simulink model "Simulink_Lab_7"  (R2025a)
settings: Solver=VariableStepAuto  StartTime=0.0  StopTime=20.0  RelTol=1e-3
libraries: spsDCMachineLib x1, spsDCVoltageSourceLib x1, sps_lib x1
settings Model: Creator=088a2  LastModifiedBy=088a2

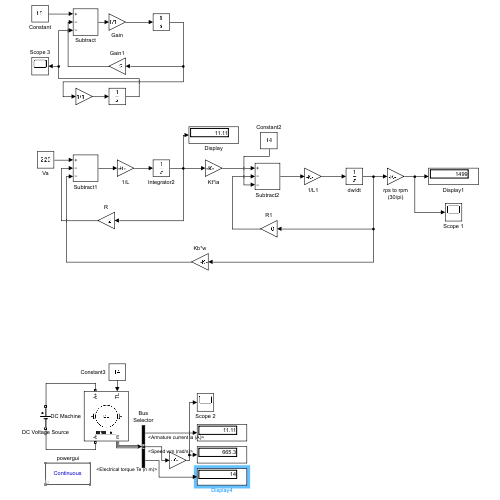
[thumbnail: Simulink's stored preview of the top-level diagram]
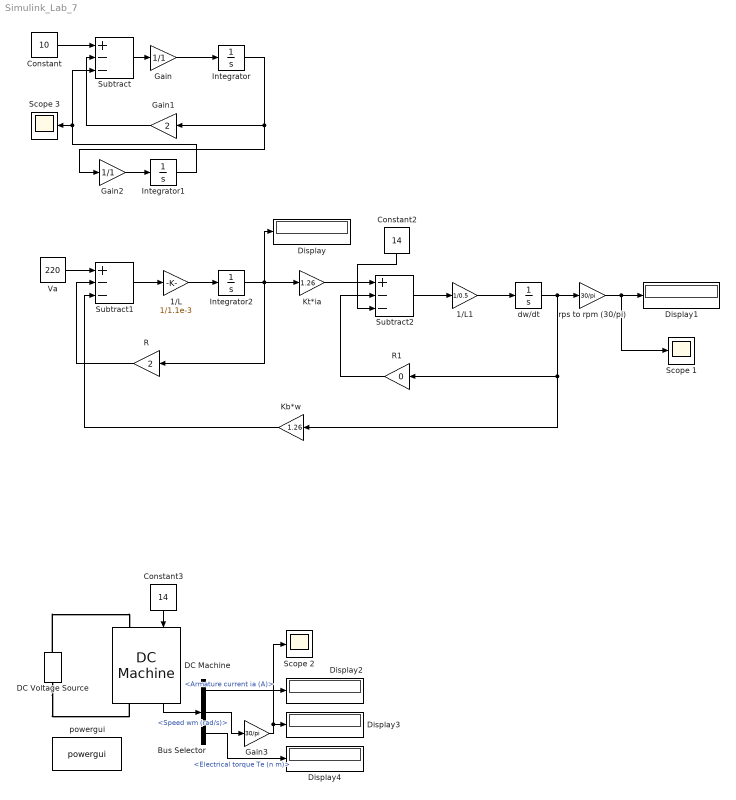
== system Simulink_Lab_7 ==
  1/L : Gain  Gain=1/1.1e-3
  1/L1 : Gain  Gain=1/0.5
  Bus Selector : BusSelector  OutputSignals=Armature current ia (A),Speed wm (rad/s),Electrical torque Te (n m)
  Constant : Constant  Value=10
  Constant2 : Constant  Value=14
  Constant3 : Constant  Value=14
  DC Machine : spsDCMachineLib/DC Machine  PresetModel=No  MechanicalLoad=Torque TL  FieldType=Permanent magnet  ShowDetailedParameters=on  MeasurementBus=off  RLa="[ 2  0.0011]"  RLf="[ 240  120]"  Laf=1.8  MachineConstant=Torque constant (N.m/A)  Ke=1.8  Kt=1.26  J=0.05  Bm=0  Tf=0  w0=1  Ifinit=1  TsPowergui=0  TsBlock=-1
  DC Voltage Source : spsDCVoltageSourceLib/DC Voltage Source  Amplitude=110  Measurements=None
  Display{,1..4} (5 alike) : Display
  Gain : Gain  Gain=1/1
  Gain1 : Gain  Gain=2
  Gain2 : Gain  Gain=1/1
  Gain3 : Gain  Gain=30/pi
  Integrator : Integrator
  Integrator1 : Integrator
  Integrator2 : Integrator
  Kb*w : Gain  Gain=1.26
  Kt*ia : Gain  Gain=1.26
  R : Gain  Gain=2
  R1 : Gain  Gain=0
  Scope 1 : Scope
      settings: Title=230929228_Mrinal_Kumar  ActiveDisplayYMinimum=-187.37365805398784  ActiveDisplayYMaximum=1686.2872524111651  YLabel=Voltage (V)
  Scope 2 : Scope
      settings: Title=230929228_Mrinal_Kumar  ActiveDisplayYMinimum=-72.596030383648909  ActiveDisplayYMaximum=747.24093799551156  YLabel=Voltage (V)
  Scope 3 : Scope
      settings: Title=230929228_Mrinal_Kumar  ActiveDisplayYMinimum=-1.2499999458908535  ActiveDisplayYMaximum=11.249999513017684  YLabel=Voltage (V)  DataLoggingVariableName=ScopeData2
  Subtract : Sum  Inputs=+--
  Subtract1 : Sum  Inputs=+--
  Subtract2 : Sum  Inputs=+--
  Va : Constant  Value=220
  dw/dt : Integrator
  powergui : sps_lib/powergui  Priority=1  SimulationMode=Continuous  SampleTime=50e-6  frequency=60  Iterations=50  frequencyindice=0  Pbase=100e6  ErrMax=1e-4  UnitsV=kV  UnitsW=MW  buscounter=0  FunctionMessages=off  echomessages=off  EnableUseOfTLC=off  CurrentSourceSwitches=off  DisableSnubberDevices=off  DisableRonSwitches=off  DisableVfSwitches=off  DisplayEquations=off  AutomaticDiscreteSolvers=off  SolverType=Tustin/Backward Euler (TBE)  Interpol=off  ExternalGateDelay=off  methode=off  Ts=100  x0status=zero  SPID=on  SwTol=0  HookPort=off  NonlinearTolerance=1e-4  nMaxIteration=100  ContinueOnMaxIteration=off  RestoreLinks=warning  ResistiveCurrentMeasurement=off  Frange=[0:2:500]  Ylog=off  Xlog=on  ShowGrid=off  save=off  variable=ZData  structure=0  ZoomFFT=off  StartTime=0.0  cycles=1  DisplayStyle=1  fundamental=60  FreqAxis=off  MaxFrequency=1000  frequencyindicesteady=1  RmsSteady=1  display=off
  rps to rpm (30/pi) : Gain  Gain=30/pi
  wires:
  Gain/1 -> Integrator/1
  Integrator/1 -> Gain2/1, Gain1/1
  Constant/1 -> Subtract/1
  Subtract/1 -> Gain/1
  Gain1/1 -> Subtract/2
  Gain2/1 -> Integrator1/1
  Integrator1/1 -> Subtract/3, Scope 3/1
  Va/1 -> Subtract1/1
  Subtract1/1 -> 1/L/1
  1/L/1 -> Integrator2/1
  Integrator2/1 -> Kt*ia/1, R/1, Display/1
  Kt*ia/1 -> Subtract2/1
  dw/dt/1 -> Kb*w/1, R1/1, rps to rpm (30/pi)/1
  rps to rpm (30/pi)/1 -> Display1/1, Scope 1/1
  Constant2/1 -> Subtract2/3
  Subtract2/1 -> 1/L1/1
  1/L1/1 -> dw/dt/1
  R1/1 -> Subtract2/2
  R/1 -> Subtract1/2
  Kb*w/1 -> Subtract1/3
  Constant3/1 -> DC Machine/1
  DC Machine/1 -> Bus Selector/1
  Bus Selector/3 -> Display4/1  "<Electrical torque Te (n m)>"
  Bus Selector/1 -> Display2/1  "<Armature current ia (A)>"
  Bus Selector/2 -> Gain3/1  "<Speed wm (rad/s)>"
  Gain3/1 -> Scope 2/1, Display3/1
  connections:
  DC Voltage Source/RConn1 -- DC Machine/LConn1
  DC Voltage Source/LConn1 -- DC Machine/RConn1
